simulink model "verify_Floor_In_mdl"  (R2016b)
settings: Solver=ode45  StartTime=0  StopTime=24*3600  MaxStep=100  RelTol=1e-3  EnableMultiTasking=on
libraries: carnot x5
settings Model: Creator=drhf  LastModifiedBy=drhf
settings DataIOCC: SaveFormat=Array  SignalLoggingSaveFormat=ModelDataLogs
settings OptimizationCC: ExpressionDepthLimit=2147483647  LifeSpan=inf
settings DebuggingCC: UnderspecifiedInitializationDetection=Classic  MergeDetectMultiDrivingBlocksExec=none  SolverPrmCheckMsg=warning  FcnCallInpInsideContextMsg=warning  StateNameClashWarn=warning  SFUnexpectedBacktrackingDiag=warning  SFNoUnconditionalDefaultTransitionDiag=warning  SFExecutionAtInitializationDiag=none
settings HardwareCC: ProdBitPerPointer=32  ProdBitPerSizeT=32  ProdBitPerPtrDiffT=32  ProdLargestAtomicFloat=None  ProdIntDivRoundTo=Undefined  ProdEndianess=Unspecified  ProdWordSize=32  ProdHWDeviceType=32-bit Generic
settings ModelReferenceCC: PropagateSignalLabelsOutOfModel=off
settings GRTTargetCC: TargetLangStandard=C89/C90 (ANSI)  GeneratePreprocessorConditionals=Disable all  CombineOutputUpdateFcns=off  GRTInterface=on
settings ConfigComp: CovMetricSettings=dw  CovHtmlReporting=on  CovSaveCumulativeToWorkspaceVar=on  CovSaveSingleToWorkspaceVar=on  CovExternalEMLEnable=off

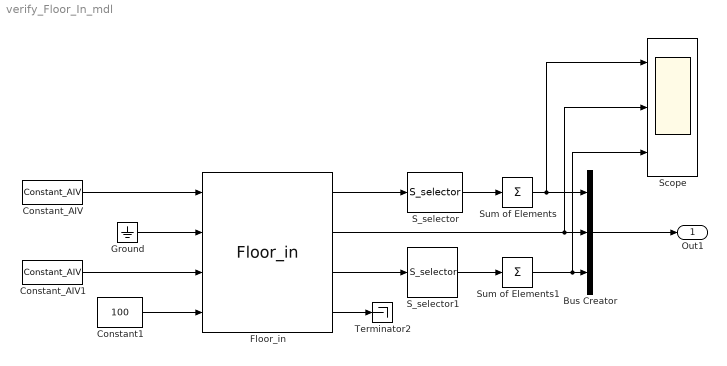
== system verify_Floor_In_mdl ==
  Bus Creator : BusCreator  Inputs=3
  Constant1 : Constant  Value=100
  Constant_AIV : carnot/Source/Ventilation/Constant_AIV  Tsens=20  Tcon=20  Trad=20  mw=0.012  mco=0.01  rhoair=1.2  cpair=1004  pair=100000  nair=0.5
  Constant_AIV1 : carnot/Source/Ventilation/Constant_AIV  Tsens=0  Tcon=0  Trad=0  mw=0.012  mco=0.01  rhoair=1.2  cpair=1004  pair=100000  nair=0.5
  Floor_in : carnot/Basic/Thermal_Models/Floor_in  wallsize=[5 5]  t0=20  d=[0.015 0.38 0.02]  cond=[1.4 0.79 0.7]  cwall=[0.28 0.28 0.28]*3600  rho=[2000 1800 1400]  misc=[.65 .65]  dactive=-1  tau=1000*3600
  Ground : Ground
  S_selector : carnot/Outputs/S_selector  e1=off  e2=off  e3=off  e4=off  e5=off  e6=off  e7=on  e8=on  e9=off  e10=off  e11=off  e12=off  e13=off
  S_selector1 : carnot/Outputs/S_selector  e1=off  e2=off  e3=off  e4=off  e5=off  e6=off  e7=on  e8=on  e9=off  e10=off  e11=off  e12=off  e13=off
  Scope : Scope  NumInputPorts=3
  Sum of Elements : Sum  Inputs=+
  Sum of Elements1 : Sum  Inputs=+
  Terminator2 : Terminator
  Out1 : Outport
  wires:
  Bus Creator/1 -> Out1/1
  Floor_in/1 -> S_selector/1
  Floor_in/3 -> S_selector1/1
  Floor_in/4 -> Terminator2/1
  Constant_AIV/1 -> Floor_in/1
  Constant_AIV1/1 -> Floor_in/3
  Constant1/1 -> Floor_in/4
  Ground/1 -> Floor_in/2
  S_selector/1 -> Sum of Elements/1
  Floor_in/2 -> Scope/2, Bus Creator/2
  S_selector1/1 -> Sum of Elements1/1
  Sum of Elements/1 -> Scope/1, Bus Creator/1
  Sum of Elements1/1 -> Scope/3, Bus Creator/3
